simulink model "channeldoc"  (Simulink 5.0)
settings: Solver=ode45  SolverMode=SingleTasking  StartTime=0.0  StopTime=inf  RelTol=1e-3
undefined symbols (not defined in the file or in its folder): slcm
libraries: commrandsrc2 x1, commchan2 x1, commsink2 x1
settings Model: Creator=ptrow  LastModifiedBy=ptrow  SaveTime=off  SaveOutput=off  AlgebraicLoopMsg=error  RTWInlineParameters=on  BooleanDataType=off  RTWOptions=-aRollThreshold=5

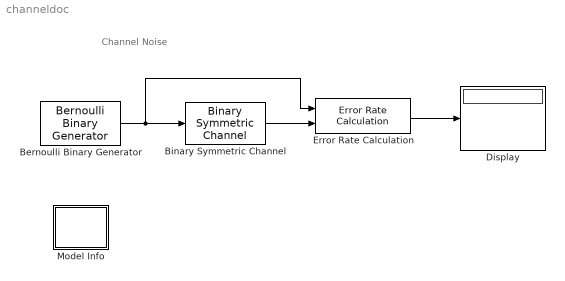
== system channeldoc ==
  note: Channel Noise
  " Display" : Display
  Bernoulli Binary Generator : commrandsrc2/Bernoulli Binary Generator  P=0.5  seed=61  Ts=1  frameBased=off  sampPerFrame=1  orient=off
  Binary Symmetric Channel : commchan2/Binary Symmetric Channel  P=0.01  s=2137  E=off
  Error Rate Calculation : commsink2/Error Rate Calculation  N=0  st_delay=0  cp_mode=Entire frame  subframe=[]  PMode=Port  WsName=ErrorVec  RsMode2=off  stop=on  numErr=100  maxBits=1e6
  Model Info : Subsystem  LoadFcn=slcm LoadBlock;  InitFcn=slcm('UpdateAllCMBlocksInThisModelInit')  mask(CMBlock){InitialSaveTempField=, InitialBlockCM=None, BlockCM=None, Frame=on, SaveTempField=, DisplayStringWithTags=Info, MaskDisplayString=Info, HorizontalTextAlignment=Center, LeftAlignmentValue=0.5, SourceBlockDiagram=channeldoc, TagMaxNumber=20, CMTag1=, CMTag2=, CMTag3=, CMTag4=, CMTag5=, CMTag6=, CMTag7=, CMTag8=, CMTag9=, CMTag10=, CMTag11=, CMTag12=, CMTag13=, CMTag14=, CMTag15=, CMTag16=, CMTag17=, CMTag18=, CMTag19=, CMTag20=}
      mask help: This block allows revision control information to be displayed within the model.
      settings: CopyFcn=slcm CopyBlock;  DeleteFcn=slcm Cancel;  PostSaveFcn=slcm('UpdateAllCMBlocksInThisModel')  NameChangeFcn=slcm Rename;  OpenFcn=commdemohelp;
      mask Display: text(str2num(LeftAlignmentValue), 0.5, MaskDisplayString, 'HorizontalAlignment', HorizontalTextAlignment)
  wires:
  Error Rate Calculation/1 -> " Display"/1
  Bernoulli Binary Generator/1 -> Error Rate Calculation/1, Binary Symmetric Channel/1
  Binary Symmetric Channel/1 -> Error Rate Calculation/2

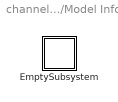
== system channeldoc/Model Info ==
  EmptySubsystem : Subsystem

== system channeldoc/Model Info/EmptySubsystem ==
